simulink model "Herman_Problema1sim"  (R2021b)
settings: Solver=VariableStepAuto  StartTime=0.0  StopTime=70.0  RelTol=1e-3
values from neighbouring files (symbols this model uses):
  A = zeros(12)    [Herman_Problema1.m]
  B = zeros(12,4)    [Herman_Problema1.m]
  C = zeros(4,12)    [Herman_Problema1.m]
  K = place(A,B,P)    [Herman_Problema1.m]
  k_bar = (C* (-A+B*K)^(-1)*B)^(-1)    [Herman_Problema1.m]
  phase = pi/2    (= 1.57079632679)    [Herman_Problema1.m]
  x_bar = [0;0;0;0;2;0;0;0;0;0;0;0]    [Herman_Problema1.m]
libraries: simulink x1
settings Model: Creator=dr.gerardocastanon  LastModifiedBy=dr.gerardocastanon

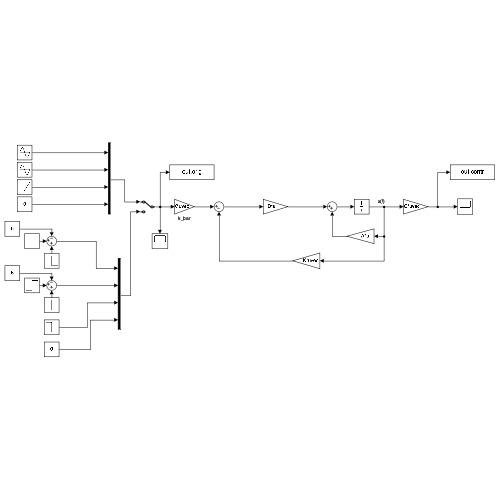
[thumbnail: Simulink's stored preview of the top-level diagram]
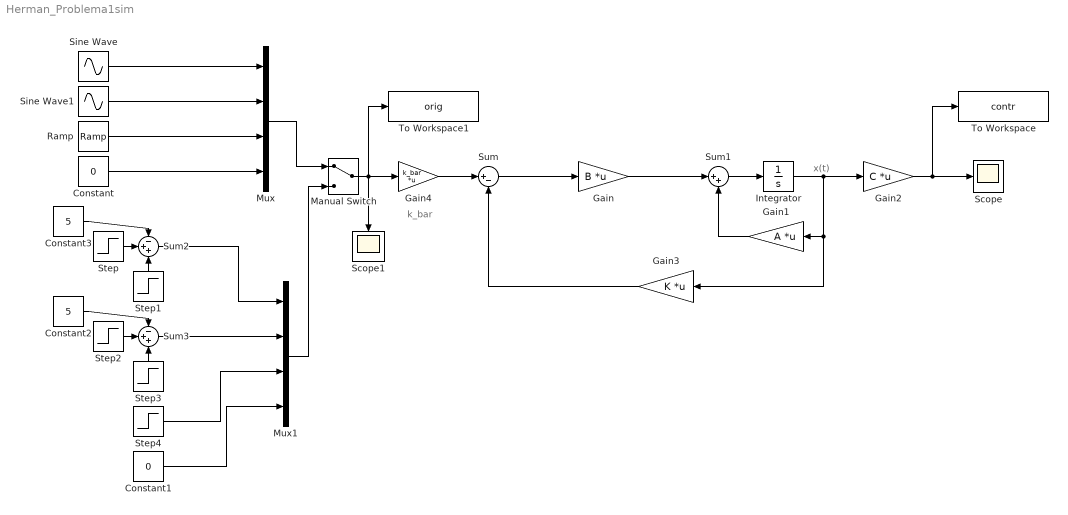
== system Herman_Problema1sim ==
  note: x(t)
  note: k_bar
  Constant : Constant  Value=0
  Constant1 : Constant  Value=0
  Constant2 : Constant  Value=5
  Constant3 : Constant  Value=5
  Gain : Gain  Gain=B  Multiplication=Matrix(K*u)
  Gain1 : Gain  Gain=A  Multiplication=Matrix(K*u)
  Gain2 : Gain  Gain=C  Multiplication=Matrix(K*u) (u vector)
  Gain3 : Gain  Gain=K  Multiplication=Matrix(K*u) (u vector)
  Gain4 : Gain  Gain=k_bar  Multiplication=Matrix(K*u) (u vector)
  Integrator : Integrator  InitialCondition=x_bar
  Manual Switch : ManualSwitch
  Mux : Mux
  Mux1 : Mux
  Ramp : simulink/Sources/Ramp  slope=0.2  start=0  InitialOutput=0
  Scope : Scope
  Scope1 : Scope
  Sine Wave : Sin  Amplitude=2  Frequency=0.2  Phase=phase  SampleTime=0
  Sine Wave1 : Sin  Amplitude=2  Frequency=0.2  SampleTime=0
  Step : Step  Time=10  After=5  SampleTime=0
  Step1 : Step  Time=30  Before=5  After=0  SampleTime=0
  Step2 : Step  Time=20  After=5  SampleTime=0
  Step3 : Step  Time=40  Before=5  After=0  SampleTime=0
  Step4 : Step  Time=50  Before=3  After=0  SampleTime=0
  Sum : Sum  Inputs=|+-
  Sum1 : Sum  Inputs=|++
  Sum2 : Sum  Inputs=-++
  Sum3 : Sum  Inputs=-++
  To Workspace : ToWorkspace  VariableName=contr  SampleTime=-1
  To Workspace1 : ToWorkspace  VariableName=orig  SampleTime=-1
  wires:
  Sine Wave/1 -> Mux/1
  Ramp/1 -> Mux/3
  Constant/1 -> Mux/4
  Mux/1 -> Manual Switch/1
  Manual Switch/1 -> To Workspace1/1, Gain4/1, Scope1/1
  Sum1/1 -> Integrator/1
  Gain3/1 -> Sum/2
  Gain/1 -> Sum1/1
  Gain1/1 -> Sum1/2
  Gain2/1 -> To Workspace/1, Scope/1
  Gain4/1 -> Sum/1
  Sine Wave1/1 -> Mux/2
  Step/1 -> Sum2/2
  Step1/1 -> Sum2/3
  Constant1/1 -> Mux1/4
  Step4/1 -> Mux1/3
  Sum2/1 -> Mux1/1
  Mux1/1 -> Manual Switch/2
  Step2/1 -> Sum3/2
  Step3/1 -> Sum3/3
  Constant2/1 -> Sum3/1
  Constant3/1 -> Sum2/1
  Sum3/1 -> Mux1/2
  Integrator/1 -> Gain3/1, Gain1/1, Gain2/1
  Sum/1 -> Gain/1
